simulink model "pid_pd_sim_umgebung"  (R2016b)
settings: Solver=FixedStepAuto  StartTime=0.0  StopTime=3  FixedStep=1e-3  RelTol=1e-3
values from neighbouring files (symbols this model uses):
  A_1 = A(1)    [playground.m]
  B_1 = B(1)    [playground.m]
undefined symbols (not defined in the file or in its folder): C_1, param, transfunc
libraries: simulink x3, simulink_extras x1
settings Model: Creator=nicol  LastModifiedBy=Fritz

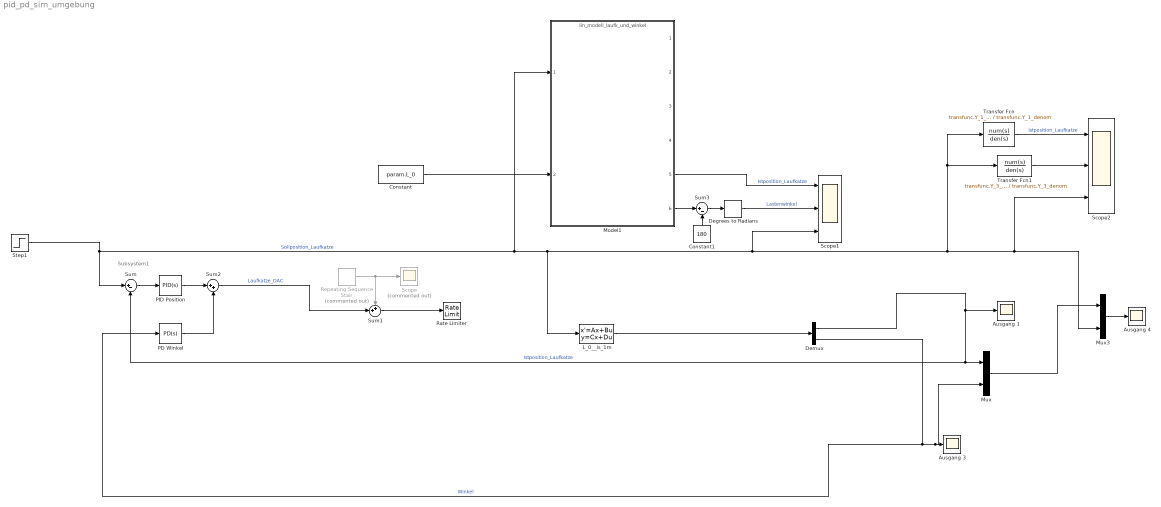
== system pid_pd_sim_umgebung ==
  note: Subsystem1
  Ausgang 1 : Scope
  Ausgang 3 : Scope
  Ausgang 4 : Scope
  Constant : Constant  Value=param.L_0
  Constant1 : Constant  Value=180
  Degrees to Radians : simulink_extras/Transformations/Degrees to Radians
  Demux : Demux  Outputs=2
  L_0__is_1m : StateSpace  A=A_1  B=B_1  C=C_1  D=[0;0]  X0=0
  Model1 : ModelReference  ModelNameDialog=lin_modell_laufk_und_winkel.slx  SimulationMode=Normal  ModelReferenceVersion=1.42
  Mux : Mux  Inputs=2
  Mux3 : Mux  Inputs=2
  PD Winkel : simulink/Continuous/PID Controller  Controller=PD  TimeDomain=Continuous-time  SampleTime=-1  IntegratorMethod=Forward Euler  FilterMethod=Forward Euler  Form=Parallel  UseFilter=on  ControllerParametersSource=internal  P=50  I=0  D=10  N=100  InitialConditionSource=internal  InitialConditionForIntegrator=0  InitialConditionForFilter=0  ExternalReset=none  LimitOutput=off  UpperSaturationLimit=inf  LowerSaturationLimit=-inf  LinearizeAsGain=on  AntiWindupMode=none  Kb=1  TrackingMode=off  Kt=1  PParamMin=[]  PParamMax=[]  IParamMin=[]  IParamMax=[]  DParamMin=[]  DParamMax=[]  NParamMin=[]  NParamMax=[]  KbParamMin=[]  KbParamMax=[]  KtParamMin=[]  KtParamMax=[]  POutMin=[]  POutMax=[]  IOutMin=[]  IOutMax=[]  DOutMin=[]  DOutMax=[]  NOutMin=[]  NOutMax=[]  KbOutMin=[]  KbOutMax=[]  KtOutMin=[]  KtOutMax=[]  IntegratorOutMin=[]  IntegratorOutMax=[]  FilterOutMin=[]  FilterOutMax=[]  SumOutMin=[]  SumOutMax=[]  SumI1OutMin=[]  SumI1OutMax=[]  SumI2OutMin=[]  SumI2OutMax=[]  SumI3OutMin=[]  SumI3OutMax=[]  SumDOutMin=[]  SumDOutMax=[]  SaturationOutMin=[]  SaturationOutMax=[]  IntegratorContinuousStateAttributes=''  IntegratorStateMustResolveToSignalObject=off  IntegratorRTWStateStorageClass=Auto  FilterContinuousStateAttributes=''  FilterStateMustResolveToSignalObject=off  FilterRTWStateStorageClass=Auto  DifferentiatorICPrevScaledInput=0  DifferentiatorOutMin=[]  DifferentiatorOutMax=[]
  PID Position : simulink/Continuous/PID Controller  Controller=PID  TimeDomain=Continuous-time  SampleTime=-1  IntegratorMethod=Forward Euler  FilterMethod=Forward Euler  Form=Parallel  UseFilter=on  ControllerParametersSource=internal  P=1  I=0.5  D=0  N=200  InitialConditionSource=internal  InitialConditionForIntegrator=0  InitialConditionForFilter=0  ExternalReset=none  LimitOutput=off  UpperSaturationLimit=inf  LowerSaturationLimit=-inf  LinearizeAsGain=on  AntiWindupMode=none  Kb=1  TrackingMode=off  Kt=1  PParamMin=[]  PParamMax=[]  IParamMin=[]  IParamMax=[]  DParamMin=[]  DParamMax=[]  NParamMin=[]  NParamMax=[]  KbParamMin=[]  KbParamMax=[]  KtParamMin=[]  KtParamMax=[]  POutMin=[]  POutMax=[]  IOutMin=[]  IOutMax=[]  DOutMin=[]  DOutMax=[]  NOutMin=[]  NOutMax=[]  KbOutMin=[]  KbOutMax=[]  KtOutMin=[]  KtOutMax=[]  IntegratorOutMin=[]  IntegratorOutMax=[]  FilterOutMin=[]  FilterOutMax=[]  SumOutMin=[]  SumOutMax=[]  SumI1OutMin=[]  SumI1OutMax=[]  SumI2OutMin=[]  SumI2OutMax=[]  SumI3OutMin=[]  SumI3OutMax=[]  SumDOutMin=[]  SumDOutMax=[]  SaturationOutMin=[]  SaturationOutMax=[]  IntegratorContinuousStateAttributes=''  IntegratorStateMustResolveToSignalObject=off  IntegratorRTWStateStorageClass=Auto  FilterContinuousStateAttributes=''  FilterStateMustResolveToSignalObject=off  FilterRTWStateStorageClass=Auto  DifferentiatorICPrevScaledInput=0  DifferentiatorOutMin=[]  DifferentiatorOutMax=[]
  Rate Limiter : RateLimiter  RisingSlewLimit=4.32  FallingSlewLimit=-4.32  SampleTimeMode=inherited
  Repeating Sequence Stair : simulink/Sources/Repeating Sequence Stair  Commented=on  OutValues=[0.2 0.3]  tsamp=1  OutMin=[]  OutMax=[]  OutDataTypeStr=double  OutputDataTypeScalingMode=double  OutDataType=fixdt(0,8)  ConRadixGroup=Best Precision: Vector-wise  OutScaling=2^-12
  Scope : Scope  Commented=on
  Scope1 : Scope  NumInputPorts=3
  Scope2 : Scope  NumInputPorts=3
  Step1 : Step  Time=0.1  SampleTime=0
  Sum : Sum  Inputs=|+-
  Sum1 : Sum  Inputs=++|
  Sum2 : Sum  Inputs=|++
  Sum3 : Sum  Inputs=|+-
  Transfer Fcn : TransferFcn  Numerator=transfunc.Y_1_numer  Denominator=transfunc.Y_1_denom
  Transfer Fcn1 : TransferFcn  Numerator=transfunc.Y_3_numer  Denominator=transfunc.Y_3_denom
  wires:
  Mux/1 -> Mux3/1
  Mux3/1 -> Ausgang 4/1
  Repeating Sequence Stair/1 -> Scope/1, Sum1/1
  Sum1/1 -> Rate Limiter/1
  Constant/1 -> Model1/2
  Sum2/1 -> Sum1/2  "Laufkatze_DAC"
  Demux/2 -> PD Winkel/1, Mux/2, Ausgang 3/1  "Winkel"
  PID Position/1 -> Sum2/1
  Sum/1 -> PID Position/1
  Demux/1 -> Mux/1, Sum/2, Ausgang 1/1  "Istposition_Laufkatze"
  Step1/1 -> Sum/1, Model1/1, L_0__is_1m/1, Transfer Fcn1/1, Transfer Fcn/1, Scope2/3, Mux3/2, Scope1/3  "Sollposition_Laufkatze"
  L_0__is_1m/1 -> Demux/1
  Model1/6 -> Sum3/1
  Constant1/1 -> Sum3/2
  Sum3/1 -> Degrees to Radians/1
  PD Winkel/1 -> Sum2/2
  Degrees to Radians/1 -> Scope1/2  "Lastenwinkel"
  Model1/5 -> Scope1/1  "Istposition_Laufkatze"
  Transfer Fcn/1 -> Scope2/1  "Istposition_Laufkatze"
  Transfer Fcn1/1 -> Scope2/2
